simulink model "OscillationSystem"  (Simulink 8.4)
settings: Solver=ode45  StartTime=0.0  StopTime=1  RelTol=1e-3
libraries: NeuroModelerLibrary x29
settings Model: Creator=Bakhshiev  LastModifiedBy=Tim
settings OptimizationCC: InitFltsAndDblsToZero=on

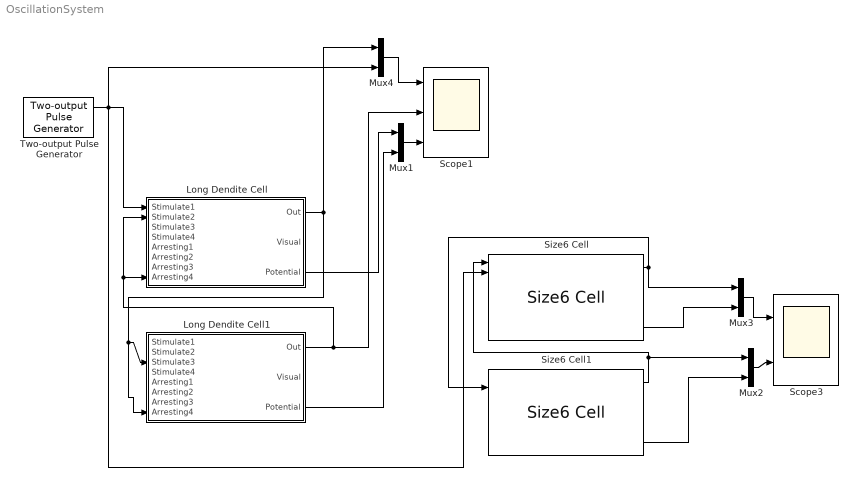
== system OscillationSystem ==
  Long Dendite Cell : Subsystem  AncestorBlock=NeuroModelerLibrary/Dendrites Cells/Long Dendite Cell
  Long Dendite Cell1 : Subsystem  AncestorBlock=NeuroModelerLibrary/Dendrites Cells/Long Dendite Cell
  Mux{1..4} (4 alike) : Mux  Inputs=2
  Scope1 : Scope  NumInputPorts=3
      settings: TimeRange=0.3271604938271605  YMin=0~0~-0.05  YMax=1~1~0.02  MaxDataPoints=5000000
  Scope3 : Scope  NumInputPorts=2
      settings: TimeRange=0.1136712749615975  YMin=-0.25~-0.25  YMax=1~1  SaveName=ScopeData2  MaxDataPoints=5000000
  Size6 Cell : NeuroModelerLibrary/Sized Cells/Size6 Cell
  Size6 Cell1 : NeuroModelerLibrary/Sized Cells/Size6 Cell
  Two-output Pulse Generator : NeuroModelerLibrary/Support/Two-output Pulse Generator  A=1  P1=200  P2=200  PW=1  ST=0.001  OOn1=0.15  OOff1=0.2  OOn2=0.25  OOff2=0.3
  wires:
  Long Dendite Cell/1(Out) -> Long Dendite Cell1/3(Stimulate3), Long Dendite Cell1/8(Arresting4), Mux4/1
  Long Dendite Cell1/1(Out) -> Scope1/2, Long Dendite Cell/8(Arresting4), Long Dendite Cell/2(Stimulate2)
  Two-output Pulse Generator/1 -> Long Dendite Cell/1(Stimulate1), Size6 Cell/2, Mux4/2
  Mux1/1 -> Scope1/3
  Long Dendite Cell/3(Potential) -> Mux1/1
  Long Dendite Cell1/3(Potential) -> Mux1/2
  Mux2/1 -> Scope3/2
  Size6 Cell1/3 -> Mux2/2
  Size6 Cell/1 -> Mux3/1, Size6 Cell1/2
  Size6 Cell1/1 -> Mux2/1, Size6 Cell/1
  Mux3/1 -> Scope3/1
  Mux4/1 -> Scope1/1
  Size6 Cell/3 -> Mux3/2

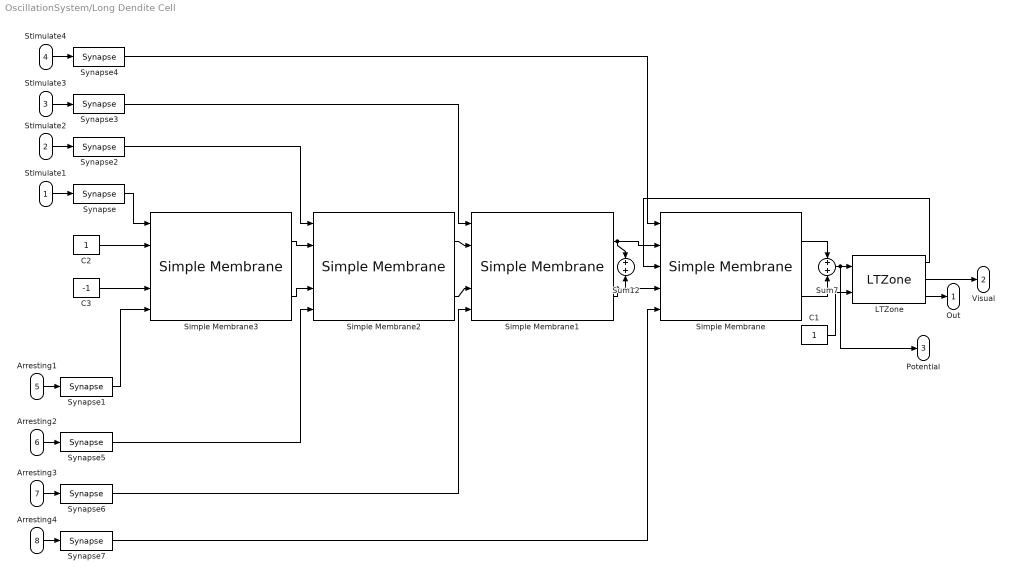
== system OscillationSystem/Long Dendite Cell ==
  Stimulate1 : Inport
  Stimulate2 : Inport  Port=2
  Stimulate3 : Inport  Port=3
  Stimulate4 : Inport  Port=4
  Arresting1 : Inport  Port=5
  Arresting2 : Inport  Port=6
  Arresting3 : Inport  Port=7
  Arresting4 : Inport  Port=8
  C1 : Constant
  C2 : Constant
  C3 : Constant  Value=-1
  LTZone : NeuroModelerLibrary/Neuron Elements/LTZone  NM=1  FB=2  IT=0.005  T=0.001
  Simple Membrane{,1..3} (4 alike) : NeuroModelerLibrary/Neuron Elements/Simple Membrane  ACm=1e-9  ARm=1e7  ECm=1e-9  ERm=1e7  ARFm=1e8  ERFm=1e8
  Sum12 : Sum  SaturateOnIntegerOverflow=on  InputSameDT=on  OutDataTypeStr=Inherit: Same as first input
  Sum7 : Sum  SaturateOnIntegerOverflow=on  InputSameDT=on  OutDataTypeStr=Inherit: Same as first input
  Synapse{,1..7} (8 alike) : NeuroModelerLibrary/Neuron Elements/Synapse  SecretionTC=0.001  DecompositionTC=0.01  ksi=1  gamma=1e8
  Out : Outport
  Visual : Outport  Port=2
  Potential : Outport  Port=3
  wires:
  Synapse7/1 -> Simple Membrane/5
  Arresting4/1 -> Synapse7/1
  Synapse6/1 -> Simple Membrane1/5
  Arresting3/1 -> Synapse6/1
  Synapse5/1 -> Simple Membrane2/5
  Arresting2/1 -> Synapse5/1
  Stimulate4/1 -> Synapse4/1
  Synapse4/1 -> Simple Membrane/1
  Stimulate3/1 -> Synapse3/1
  Stimulate2/1 -> Synapse2/1
  Synapse2/1 -> Simple Membrane2/1
  C2/1 -> Simple Membrane3/2
  C3/1 -> Simple Membrane3/4
  Synapse1/1 -> Simple Membrane3/5
  Simple Membrane3/2 -> Simple Membrane2/4
  Simple Membrane3/1 -> Simple Membrane2/2
  Simple Membrane2/2 -> Simple Membrane1/4
  Simple Membrane2/1 -> Simple Membrane1/2
  LTZone/2 -> Visual/1
  LTZone/3 -> Out/1
  C1/1 -> LTZone/2
  Stimulate1/1 -> Synapse/1
  Arresting1/1 -> Synapse1/1
  Simple Membrane1/1 -> Simple Membrane/2, Sum12/1
  Simple Membrane1/2 -> Simple Membrane/4, Sum12/2
  Sum7/1 -> LTZone/1, Potential/1
  LTZone/1 -> Simple Membrane/3
  Simple Membrane/1 -> Sum7/1
  Simple Membrane/2 -> Sum7/2
  Synapse3/1 -> Simple Membrane1/1
  Synapse/1 -> Simple Membrane3/1

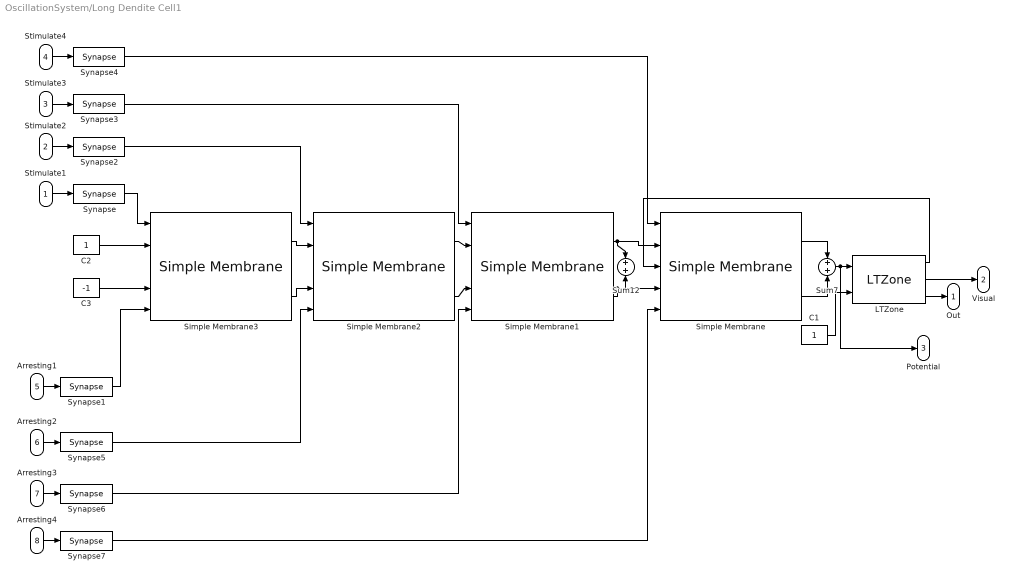
== system OscillationSystem/Long Dendite Cell1 ==
  Stimulate1 : Inport
  Stimulate2 : Inport  Port=2
  Stimulate3 : Inport  Port=3
  Stimulate4 : Inport  Port=4
  Arresting1 : Inport  Port=5
  Arresting2 : Inport  Port=6
  Arresting3 : Inport  Port=7
  Arresting4 : Inport  Port=8
  C1 : Constant
  C2 : Constant
  C3 : Constant  Value=-1
  LTZone : NeuroModelerLibrary/Neuron Elements/LTZone  NM=1  FB=2  IT=0.005  T=0.001
  Simple Membrane{,1..3} (4 alike) : NeuroModelerLibrary/Neuron Elements/Simple Membrane  ACm=1e-9  ARm=1e7  ECm=1e-9  ERm=1e7  ARFm=1e8  ERFm=1e8
  Sum12 : Sum  SaturateOnIntegerOverflow=on  InputSameDT=on  OutDataTypeStr=Inherit: Same as first input
  Sum7 : Sum  SaturateOnIntegerOverflow=on  InputSameDT=on  OutDataTypeStr=Inherit: Same as first input
  Synapse{,1..7} (8 alike) : NeuroModelerLibrary/Neuron Elements/Synapse  SecretionTC=0.001  DecompositionTC=0.01  ksi=1  gamma=1e8
  Out : Outport
  Visual : Outport  Port=2
  Potential : Outport  Port=3
  wires:
  Synapse7/1 -> Simple Membrane/5
  Arresting4/1 -> Synapse7/1
  Synapse6/1 -> Simple Membrane1/5
  Arresting3/1 -> Synapse6/1
  Synapse5/1 -> Simple Membrane2/5
  Arresting2/1 -> Synapse5/1
  Stimulate4/1 -> Synapse4/1
  Synapse4/1 -> Simple Membrane/1
  Stimulate3/1 -> Synapse3/1
  Synapse3/1 -> Simple Membrane1/1
  Stimulate2/1 -> Synapse2/1
  Synapse2/1 -> Simple Membrane2/1
  Synapse/1 -> Simple Membrane3/1
  C2/1 -> Simple Membrane3/2
  C3/1 -> Simple Membrane3/4
  Synapse1/1 -> Simple Membrane3/5
  Simple Membrane3/2 -> Simple Membrane2/4
  Simple Membrane3/1 -> Simple Membrane2/2
  Simple Membrane2/2 -> Simple Membrane1/4
  Simple Membrane2/1 -> Simple Membrane1/2
  LTZone/2 -> Visual/1
  LTZone/3 -> Out/1
  C1/1 -> LTZone/2
  Stimulate1/1 -> Synapse/1
  Arresting1/1 -> Synapse1/1
  Simple Membrane1/1 -> Simple Membrane/2, Sum12/1
  Simple Membrane1/2 -> Simple Membrane/4, Sum12/2
  Sum7/1 -> LTZone/1, Potential/1
  LTZone/1 -> Simple Membrane/3
  Simple Membrane/1 -> Sum7/1
  Simple Membrane/2 -> Sum7/2
